simulink model "mcb_pmsm_foc_qep_f28035"  (R2021b)
settings: Solver=FixedStepDiscrete  StartTime=0.0  StopTime=8  RelTol=1e-3  EnableMultiTasking=on
InitFcn:
  | mcb_pmsm_foc_qep_f28035_data
values from neighbouring files (symbols this model uses):
  inverter = mcb_SetInverterParameters('BoostXL-DRV8305')    [mcb_pmsm_foc_dual_f28379d_data.m]    (also in mcb_pmsm_foc_dual_f28379d_datascript.m; mcb_pmsm_foc_f280049C_data.m; mcb_pmsm_foc_f28335_data.m = mcb_SetInverterParameters('DRV8312-C2-KIT'); mcb_pmsm_foc_hall_f28035_data.m = mcb_SetInverterParameters('DRV8312-C2-KIT'))
  PI_params = mcb.internal.SetControllerParameters(pmsm,inverter,PU_System,T_pwm,2*Ts,Ts_speed)    [mcb_pmsm_foc_dual_f28379d_data.m]    (also in mcb_pmsm_foc_dual_f28379d_datascript.m; mcb_pmsm_foc_f280049C_data.m = mcb.internal.SetControllerParameters(pmsm,inverter,PU_System; mcb_pmsm_foc_f28335_data.m = mcb.internal.SetControllerParameters(pmsm,inverter,PU_System; mcb_pmsm_foc_hall_f28035_data.m = mcb.internal.SetControllerParameters(pmsm,inverter,PU_System)
  pmsm = struct    [c28335_pmsmfoc_data.m]    (also in mcb_pmsm_foc_dual_f28379d_data.m = mcb_SetPMSMMotorParameters('Teknic2310P'); mcb_pmsm_foc_dual_f28379d_datascript.m = mcb_SetPMSMMotorParameters('Teknic2310P'); mcb_pmsm_foc_f280049C_data.m = mcb_SetPMSMMotorParameters('BLY171D'); mcb_pmsm_foc_f28335_data.m = mcb_SetPMSMMotorParameters('BLY171D'))
  target = mcb_SetProcessorDetails('F28379D',PWM_frequency)    [mcb_pmsm_foc_dual_f28379d_data.m]    (also in mcb_pmsm_foc_dual_f28379d_datascript.m; mcb_pmsm_foc_f280049C_data.m = mcb_SetProcessorDetails('F280049C',PWM_frequency); mcb_pmsm_foc_f28335_data.m = mcb_SetProcessorDetails('F28335',PWM_frequency); mcb_pmsm_foc_hall_f28035_data.m = mcb_SetProcessorDetails('F28035',PWM_frequency))
  Ts_motor = T_pwm/2    (= 2.5e-05)    [mcb_pmsm_foc_dual_f28379d_data.m]    (also in mcb_pmsm_foc_dual_f28379d_datascript.m; mcb_pmsm_foc_f280049C_data.m; mcb_pmsm_foc_f28335_data.m; mcb_pmsm_foc_hall_f28035_data.m)
  Ts_simulink = T_pwm/2    (= 2.5e-05)    [mcb_pmsm_foc_dual_f28379d_data.m]    (also in mcb_pmsm_foc_dual_f28379d_datascript.m; mcb_pmsm_foc_f280049C_data.m; mcb_pmsm_foc_f28335_data.m; mcb_pmsm_foc_hall_f28035_data.m)
undefined symbols (not defined in the file or in its folder): Down, GPTRIP1SEL, GPTRIP2SEL, TZ1, TZ2, Up
libraries: simulink x6, c2802xlib x5, c2803xlib x3, c280xlib x3, demo_controls x1, c2000lib x1, mcbplantlib x1, mcbcontrolslib x1, autolibpmsmexterior x1
(part 2 of 2)

== system mcb_pmsm_foc_qep_f28035/Embedded Processor/Serial Receive/Simulation/Parse ==
  Enable_PWM : Inport
  Debug_signals : Inport  Port=2
  Bitwise Operator : simulink/Logic and Bit Operations/Bitwise Operator  logicop=AND  UseBitMask=on  BitMask=hex2dec('0001')  BitMaskRealWorld=Stored Integer
  Bitwise Operator1 : simulink/Logic and Bit Operations/Bitwise Operator  logicop=AND  UseBitMask=on  BitMask=hex2dec('00F0')  BitMaskRealWorld=Stored Integer
  Shift Arithmetic1 : ArithShift  BitShiftNumber=-4
  Sum : Sum  Inputs=|++
  Data : Outport
  wires:
  Bitwise Operator/1 -> Sum/1
  Debug_signals/1 -> Shift Arithmetic1/1
  Sum/1 -> Data/1
  Shift Arithmetic1/1 -> Bitwise Operator1/1
  Enable_PWM/1 -> Bitwise Operator/1
  Bitwise Operator1/1 -> Sum/2

== system mcb_pmsm_foc_qep_f28035/Inverter and Motor - Plant Model/Simulation/Sensor_Measurements/Get_PU  ==
  rad : Inport
  Constant2 : Constant  Value=2*pi  OutDataTypeStr=single  SampleTime=-1
  Get_PU : Gain  Gain=1/(2*pi)  RndMeth=Simplest  OutDataTypeStr=Inherit: Same as input
  Mod : Math  Operator=mod  SaturateOnIntegerOverflow=on
  PU : Outport  VectorParamsAs1DForOutWhenUnconnected=off
  wires:
  rad/1 -> Mod/1
  Constant2/1 -> Mod/2
  Mod/1 -> Get_PU/1
  Get_PU/1 -> PU/1

== system mcb_pmsm_foc_qep_f28035/Inverter and Motor - Plant Model/Simulation/Sensor_Measurements/Wrap ==
  in : Inport
  Constant2 : Constant  OutDataTypeStr=single  SampleTime=-1
  Mod : Math  Operator=mod  SaturateOnIntegerOverflow=on
  out : Outport  VectorParamsAs1DForOutWhenUnconnected=off
  wires:
  in/1 -> Mod/1
  Constant2/1 -> Mod/2
  Mod/1 -> out/1

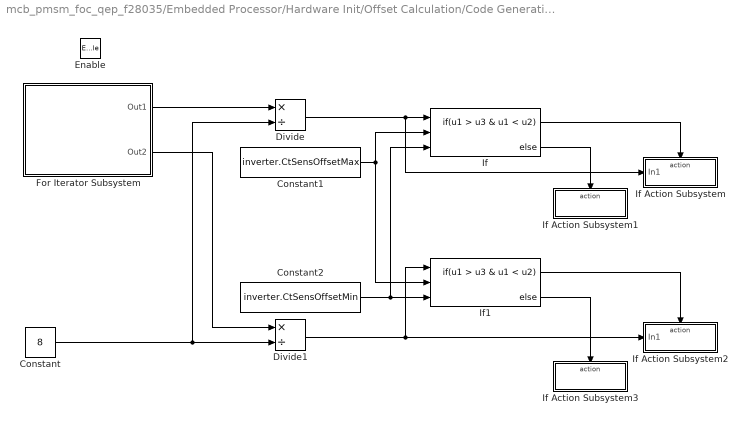
== system mcb_pmsm_foc_qep_f28035/Embedded Processor/Hardware Init/Offset Calculation/Code Generation/Calculate ADC Offset  ==
  Enable : EnablePort
  Constant : Constant  Value=8
  Constant1 : Constant  Value=inverter.CtSensOffsetMax  OutDataTypeStr=Inherit: Inherit via back propagation
  Constant2 : Constant  Value=inverter.CtSensOffsetMin  OutDataTypeStr=Inherit: Inherit via back propagation
  Divide : Product  Inputs=*/  OutDataTypeStr=uint16
  Divide1 : Product  Inputs=*/  OutDataTypeStr=uint16
  For Iterator Subsystem : Subsystem  TreatAsAtomicUnit=on
  If : If  NumInputs=3  IfExpression=u1 > u3 & u1 < u2
  If Action Subsystem : Subsystem  TreatAsAtomicUnit=on
  If Action Subsystem1 : Subsystem  TreatAsAtomicUnit=on
  If Action Subsystem2 : Subsystem  TreatAsAtomicUnit=on
  If Action Subsystem3 : Subsystem  TreatAsAtomicUnit=on
  If1 : If  NumInputs=3  IfExpression=u1 > u3 & u1 < u2
  wires:
  If1/2 -> If Action Subsystem3/Action
  Constant1/1 -> If/2, If1/2
  If1/1 -> If Action Subsystem2/Action
  If/2 -> If Action Subsystem1/Action
  If/1 -> If Action Subsystem/Action
  For Iterator Subsystem/1(Out1) -> Divide/1
  Constant2/1 -> If/3, If1/3
  For Iterator Subsystem/2(Out2) -> Divide1/1
  Divide1/1 -> If Action Subsystem2/1(In1), If1/1
  Constant/1 -> Divide1/2, Divide/2
  Divide/1 -> If Action Subsystem/1(In1), If/1

== system mcb_pmsm_foc_qep_f28035/Embedded Processor/Hardware Init/Offset Calculation/Code Generation/DRV Enable ==
  In1 : Inport
  Digital Output1 : c2803xlib/Digital Output  GPIO_Number=GPIO0~GPIO7  GPIO_Bit0=off  GPIO_BIT0_Toggle=off  GPIO_Bit1=on  GPIO_BIT1_Toggle=off  GPIO_Bit2=off  GPIO_BIT2_Toggle=off  GPIO_Bit3=on  GPIO_BIT3_Toggle=off  GPIO_Bit4=off  GPIO_BIT4_Toggle=off  GPIO_Bit5=on  GPIO_BIT5_Toggle=off  GPIO_Bit6=off  GPIO_BIT6_Toggle=off  GPIO_Bit7=off  GPIO_BIT7_Toggle=off
      settings: SourceProductBaseCode=TIC2000
  Mux : Mux  Inputs=3
  wires:
  Mux/1 -> Digital Output1/1
  In1/1 -> Mux/3, Mux/2, Mux/1

== system mcb_pmsm_foc_qep_f28035/Embedded Processor/Hardware Init/Offset Calculation/Code Generation/Default ADC Offset ==
  Enable : EnablePort
  Constant : Constant  Value=inverter.CtSensAOffset  OutDataTypeStr=Inherit: Inherit via back propagation
  Constant1 : Constant  Value=inverter.CtSensBOffset  OutDataTypeStr=Inherit: Inherit via back propagation
  Data Store Write1 : DataStoreWrite  DataStoreName=IaOffset  IndexOptions=Index vector (dialog)  Indices=1  OutputSizes=1
  Data Store Write2 : DataStoreWrite  DataStoreName=IbOffset  IndexOptions=Index vector (dialog)  Indices=1  OutputSizes=1
  wires:
  Constant/1 -> Data Store Write1/1
  Constant1/1 -> Data Store Write2/1

== system mcb_pmsm_foc_qep_f28035/Embedded Processor/Hardware Init/Offset Calculation/Code Generation/Calculate ADC Offset /For Iterator Subsystem ==
  Demux : Demux  Outputs=2
  For Iterator : ForIterator  IterationLimit=16  IterationVariableDataType=uint16
  IA/IB Measurement : c2802xlib/ADC  blkParamProc=C2000  ADCModule=1  samplingMode=Simultaneous sample mode  ADCResolution=12-bit (Single-ended input)  useSOC1=SOC0  useSOC2=SOC2_SOC3  SOCAcquisitionWindow=7  SOCTriggerSource=Software  SOCInterruptTrigger=No ADCINT  Ts=-1  dType=uint16  postInterrupt=off  interruptSel=ADCINT1  ADCINTContinuous=on  endma=off  chdma=1  conv1=ADCINA0  conv2=ADCINA1 and ADCINB1  conv1_Type4=ADCIN0  conv2_Type4=ADCIN0 and ADCIN1
  If : If  IfExpression=u1 > 8  ShowElse=off
  If Action Subsystem : Subsystem  TreatAsAtomicUnit=on
  Out1 : Outport
  Out2 : Outport  Port=2
  wires:
  For Iterator/1 -> If/1
  If Action Subsystem/1(Out1) -> Out1/1
  If Action Subsystem/2(Out2) -> Out2/1
  If/1 -> If Action Subsystem/Action
  Demux/1 -> If Action Subsystem/1(In1)
  Demux/2 -> If Action Subsystem/2(In2)
  IA/IB Measurement/1 -> Demux/1

== system mcb_pmsm_foc_qep_f28035/Embedded Processor/Hardware Init/Offset Calculation/Code Generation/Calculate ADC Offset /If Action Subsystem ==
  In1 : Inport
  Action Port : ActionPort
  Data Store Write1 : DataStoreWrite  DataStoreName=IaOffset  IndexOptions=Index vector (dialog)  Indices=1  OutputSizes=1
  wires:
  In1/1 -> Data Store Write1/1

== system mcb_pmsm_foc_qep_f28035/Embedded Processor/Hardware Init/Offset Calculation/Code Generation/Calculate ADC Offset /If Action Subsystem1 ==
  Action Port : ActionPort
  Constant : Constant  Value=inverter.CtSensAOffset  OutDataTypeStr=Inherit: Inherit via back propagation
  Data Store Write1 : DataStoreWrite  DataStoreName=IaOffset  IndexOptions=Index vector (dialog)  Indices=1  OutputSizes=1
  wires:
  Constant/1 -> Data Store Write1/1

== system mcb_pmsm_foc_qep_f28035/Embedded Processor/Hardware Init/Offset Calculation/Code Generation/Calculate ADC Offset /If Action Subsystem2 ==
  In1 : Inport
  Action Port : ActionPort
  Data Store Write2 : DataStoreWrite  DataStoreName=IbOffset  IndexOptions=Index vector (dialog)  Indices=1  OutputSizes=1
  wires:
  In1/1 -> Data Store Write2/1

== system mcb_pmsm_foc_qep_f28035/Embedded Processor/Hardware Init/Offset Calculation/Code Generation/Calculate ADC Offset /If Action Subsystem3 ==
  Action Port : ActionPort
  Constant1 : Constant  Value=inverter.CtSensBOffset  OutDataTypeStr=Inherit: Inherit via back propagation
  Data Store Write2 : DataStoreWrite  DataStoreName=IbOffset  IndexOptions=Index vector (dialog)  Indices=1  OutputSizes=1
  wires:
  Constant1/1 -> Data Store Write2/1

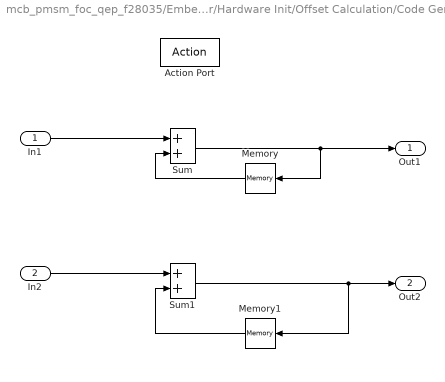
== system mcb_pmsm_foc_qep_f28035/Embedded Processor/Hardware Init/Offset Calculation/Code Generation/Calculate ADC Offset /For Iterator Subsystem/If Action Subsystem ==
  In1 : Inport
  In2 : Inport  Port=2
  Action Port : ActionPort
  Memory : Memory  InheritSampleTime=on
  Memory1 : Memory  InheritSampleTime=on
  Sum : Sum
  Sum1 : Sum
  Out1 : Outport
  Out2 : Outport  Port=2
  wires:
  In1/1 -> Sum/1
  Sum/1 -> Out1/1, Memory/1
  In2/1 -> Sum1/1
  Memory/1 -> Sum/2
  Sum1/1 -> Out2/1, Memory1/1
  Memory1/1 -> Sum1/2
